simulink model "engine_cl_tuned"  (R2018b)
settings: Solver=VariableStepAuto  StartTime=0  StopTime=options.T_train  MaxStep=0.01  RelTol=1e-3  EnableMultiTasking=on
PreLoadFcn:
  | Kp=0.0055;
  | Ki=0.0131;
  | Kd=3.3894e-004;
  | N=9.9135;
model workspace (MAT data in the model file):
  p = [-7.82997288351e-05; 0.181210895977; -0.072497134344; 0.000486358314052; 0.0361674637937]
undefined symbols (not defined in the file or in its folder): options
libraries: neural x132, simulink x4
(part 6 of 6)

== system engine_cl_tuned/NN_cex_1/Layer 3/Delays 1 ==
  "p{3}" : Inport  PortDimensions=30
      mask Display: e = 0.06;c1 = [120 230 180]/255;c2 = ([120 230 180]+0)/(256+128);c3 = ([120 230 180]+128)/(256+128);patch([0 1 1 0],[0 0 1 1],c1);patch([0 1 1 1-e 1-e 0+e],[0 0 1 1-e 0+e 0+e],c2);patch([0 0 1 1-e 0+e 0+e],[0 1 1 1-e 1-e 0+e],c3);plot([0 1 1 0 0],[0 0 1 1 0]);
  mux : Mux  Inputs=1
      mask Display: e = 0.06;c1 = [120 150 230]/255;c2 = ([120 150 230]+0)/383;c3 = ([120 150 230]+128)/383;patch([0 1 1 0],[0 0 1 1],c1);patch([0 1 1 1-e 1-e 0+e],[0 0 1 1-e 0+e 0+e],c2);patch([0 0 1 1-e 0+e 0+e],[0 1 1 1-e 1-e 0+e],c3);plot([0 1 1 0 0],[0 0 1 1 0]);disp('Mux')
  "pd{3,2}" : Outport
      mask Display: e = 0.06;c1 = [120 230 180]/255;c2 = ([120 230 180]+0)/(256+128);c3 = ([120 230 180]+128)/(256+128);patch([0 1 1 0],[0 0 1 1],c1);patch([0 1 1 1-e 1-e 0+e],[0 0 1 1-e 0+e 0+e],c2);patch([0 0 1 1-e 0+e 0+e],[0 1 1 1-e 1-e 0+e],c3);plot([0 1 1 0 0],[0 0 1 1 0]);
  wires:
  "p{3}"/1 -> mux/1
  mux/1 -> "pd{3,2}"/1

== system engine_cl_tuned/NN_cex_1/Layer 3/LW{3,2} ==
  "ad{3,2}" : Inport  PortDimensions=30
      mask Display: e = 0.06;c1 = [120 230 180]/255;c2 = ([120 230 180]+0)/(256+128);c3 = ([120 230 180]+128)/(256+128);patch([0 1 1 0],[0 0 1 1],c1);patch([0 1 1 1-e 1-e 0+e],[0 0 1 1-e 0+e 0+e],c2);patch([0 0 1 1-e 0+e 0+e],[0 1 1 1-e 1-e 0+e],c3);plot([0 1 1 0 0],[0 0 1 1 0]);
  "IW{3,2}(1,:)'" : Constant  Value=[-0.05585272353059651806450602862241794355213642120361328125;0.09223152263494603653182224434203817509114742279052734375;0.61816465960493616194071364589035511016845703125;-0.574664768951687943143724623951129615306854248046875;-0.40275843015105861066871284492663107812404632568359375;0.90766911071132627686353089302428998053073883056640625;-0.2716239584167994269847667965223081409931182861328125;-0.773180427101555434177271308726631104946136474609375;-0.237913795169213682090258998869103379547595977783203125;0.7805301361368599533108181276475079357624053955078125;-0.055675393872570665132482048420570208691060543060302734375;0.63817697881333146359139618652989156544208526611328125;-0.73282669401900080163869688476552255451679229736328125;0.97202785870217833785744687702390365302562713623046875;-0.263669215077264318392025188586558215320110321044921875;0.397746749932118059955854505460592918097972869873046875;-0.51852654200736825185202860666322521865367889404296875;0.58665753887857963189134125059354119002819061279296875;-0.719068086029560848970731967710889875888824462890625;-0.6090759721022613870644590861047618091106414794921875;0.12230193905379919960818568824834073893725872039794921875;0.421097653063960353225780863795080222189426422119140625;-0.72636663509911059133372646101634018123149871826171875;0.8571409070790594331157308261026628315448760986328125;0.26848233336055293829502943481202237308025360107421875;-0.83187954590848300906458234749152325093746185302734375;0.291448643609701740775363987268065102398395538330078125;-0.091291234566807155648149318949435837566852569580078125;0.28790720091232291366623030626215040683746337890625;-0.86123712386536610541298841781099326908588409423828125]
      mask Display: e = 0.06;c1 = [120 150 230]/255;c2 = ([120 150 230]+0)/383;c3 = ([120 150 230]+128)/383;patch([0 1 1 0],[0 0 1 1],c1);patch([0 1 1 1-e 1-e 0+e],[0 0 1 1-e 0+e 0+e],c2);patch([0 0 1 1-e 0+e 0+e],[0 1 1 1-e 1-e 0+e],c3);plot([0 1 1 0 0],[0 0 1 1 0]);disp('weights');
  Mux : Mux  Inputs=1
      mask Display: e = 0.06;c1 = [120 150 230]/255;c2 = ([120 150 230]+0)/383;c3 = ([120 150 230]+128)/383;patch([0 1 1 0],[0 0 1 1],c1);patch([0 1 1 1-e 1-e 0+e],[0 0 1 1-e 0+e 0+e],c2);patch([0 0 1 1-e 0+e 0+e],[0 1 1 1-e 1-e 0+e],c3);plot([0 1 1 0 0],[0 0 1 1 0]);disp('Mux');
  dotprod1 : neural/Weight Functions/dotprod
  "lz{3,2}" : Outport
      mask Display: e = 0.06;c1 = [120 230 180]/255;c2 = ([120 230 180]+0)/(256+128);c3 = ([120 230 180]+128)/(256+128);patch([0 1 1 0],[0 0 1 1],c1);patch([0 1 1 1-e 1-e 0+e],[0 0 1 1-e 0+e 0+e],c2);patch([0 0 1 1-e 0+e 0+e],[0 1 1 1-e 1-e 0+e],c3);plot([0 1 1 0 0],[0 0 1 1 0]);
  wires:
  "IW{3,2}(1,:)'"/1 -> dotprod1/1
  "ad{3,2}"/1 -> dotprod1/2
  dotprod1/1 -> Mux/1
  Mux/1 -> "lz{3,2}"/1
